simulink model "model2_observable"  (R2024a)
settings: Solver=VariableStepAuto  StartTime=0.0  StopTime=10.0  RelTol=1e-3
settings Model: Creator=Professional  LastModifiedBy=Professional

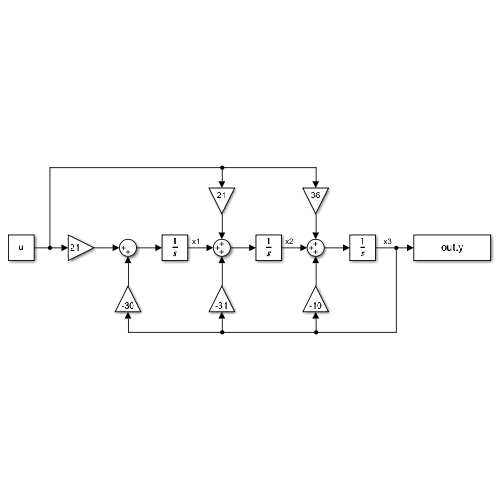
[thumbnail: Simulink's stored preview of the top-level diagram]
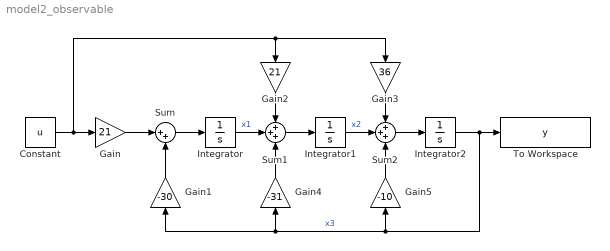
== system model2_observable ==
  Constant : Constant  Value=u  SampleTime=0.0001
  Gain : Gain  Gain=21
  Gain1 : Gain  Gain=-30
  Gain2 : Gain  Gain=21
  Gain3 : Gain  Gain=36
  Gain4 : Gain  Gain=-31
  Gain5 : Gain  Gain=-10
  Integrator : Integrator
  Integrator1 : Integrator
  Integrator2 : Integrator
  Sum : Sum  Inputs=|++
  Sum1 : Sum  Inputs=+++
  Sum2 : Sum  Inputs=+++
  To Workspace : ToWorkspace  VariableName=y  SaveFormat=Timeseries  SampleTime=-1
  wires:
  Constant/1 -> Gain3/1, Gain2/1, Gain/1
  Gain/1 -> Sum/1
  Gain1/1 -> Sum/2
  Sum/1 -> Integrator/1
  Integrator/1 -> Sum1/2  "x1"
  Gain2/1 -> Sum1/1
  Sum1/1 -> Integrator1/1
  Gain3/1 -> Sum2/1
  Integrator1/1 -> Sum2/2  "x2"
  Gain4/1 -> Sum1/3
  Gain5/1 -> Sum2/3
  Sum2/1 -> Integrator2/1
  Integrator2/1 -> To Workspace/1, Gain1/1, Gain4/1, Gain5/1  "x3"
